simulink model "mov_avg_try"  (R2022b)
settings: Solver=VariableStepAuto  StartTime=0.0  StopTime=1  RelTol=1e-3
libraries: simulink_extras x1, spsEdgeDetectorLib x1, spsSampleandHoldLib x1
settings Model: Creator=srikri  LastModifiedBy=srikri

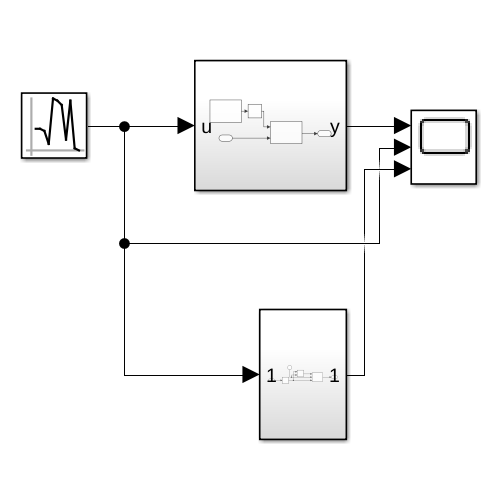
[thumbnail: Simulink's stored preview of the top-level diagram]
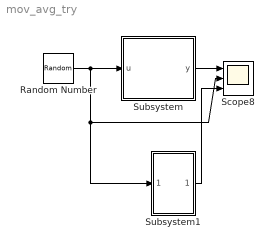
== system mov_avg_try ==
  Random Number : RandomNumber  SampleTime=0.1
  Scope8 : Scope  NumInputPorts=3
  Subsystem : Subsystem
  Subsystem1 : Subsystem
  wires:
  Random Number/1 -> Subsystem1/1(In1), Scope8/2, Subsystem/1(u)
  Subsystem/1(y) -> Scope8/1
  Subsystem1/1(Out1) -> Scope8/3

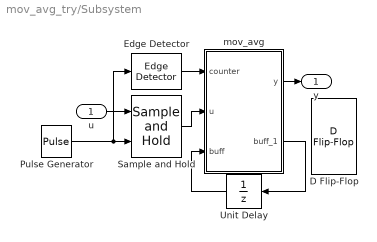
== system mov_avg_try/Subsystem ==
  u : Inport
  D Flip-Flop : simulink_extras/Flip Flops/D Flip-Flop
  Edge Detector : spsEdgeDetectorLib/Edge Detector  model=Rising  ic=0  Ts=0
      settings: LibrarySourceBlock=sps_lib/Control/Edge Detector
  Pulse Generator : DiscretePulseGenerator  PulseType=Time based  Period=1/1e3  PulseWidth=5
  Sample and Hold : spsSampleandHoldLib/Sample and Hold  ic=0  Ts=0
      settings: LibrarySourceBlock=|
      | sps_lib/Control/Sample and
      | Hold
  Unit Delay : UnitDelay  SampleTime=-1  HasFrameUpgradeWarning=on
  mov_avg : MATLAB Function  TreatAsAtomicUnit=on
  y : Outport
  wires:
  mov_avg/1(y) -> y/1
  u/1 -> Sample and Hold/1
  Edge Detector/1 -> mov_avg/1(counter)
  Sample and Hold/1 -> mov_avg/2(u)
  Pulse Generator/1 -> Edge Detector/1, Sample and Hold/2
  mov_avg/2(buff_1) -> Unit Delay/1
  Unit Delay/1 -> mov_avg/3(buff)

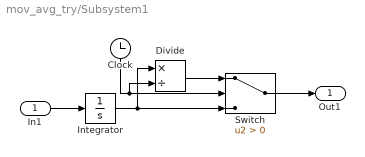
== system mov_avg_try/Subsystem1 ==
  In1 : Inport
  Clock : Clock
  Divide : Product  Inputs=*/
  Integrator : Integrator
  Switch : Switch  Criteria=u2 > Threshold  SaturateOnIntegerOverflow=off  InputSameDT=off
  Out1 : Outport
  wires:
  Divide/1 -> Switch/1
  Integrator/1 -> Switch/3, Divide/1
  Clock/1 -> Switch/2, Divide/2
  In1/1 -> Integrator/1
  Switch/1 -> Out1/1

== matlab function mov_avg_try/Subsystem/mov_avg ==
  data: counter input; u input; y output; buff input; buff_1 output
function [y,buff_1] = fcn(counter, u, buff)
    if counter
        for i = 1:9
            buff(i+1) = buff(i);
        end
        buff(1) = u;
        y = sum(buff)/10;
    else
        y = sum(buff)/10;
    end
buff_1 = buff;
end
